simulink subsystem "PID"  (R2024b)
settings: Solver=VariableStepAuto  StartTime=0.0  StopTime=10.0  RelTol=1e-3
values from neighbouring files (symbols this model uses):
  Kd = 1.84    [Controller_PIDTuning.m]
  Ki = 98    [Controller_PIDTuning.m]
  Kp = 32.3    [Controller_PIDTuning.m]
  Kw = 1/Tw    (= 5.88235294118)    [Controller_PIDTuning.m]
  TL = b / wc    [Controller_PIDTuning.m]
settings Model: Creator=Utente  LastModifiedBy=Buton

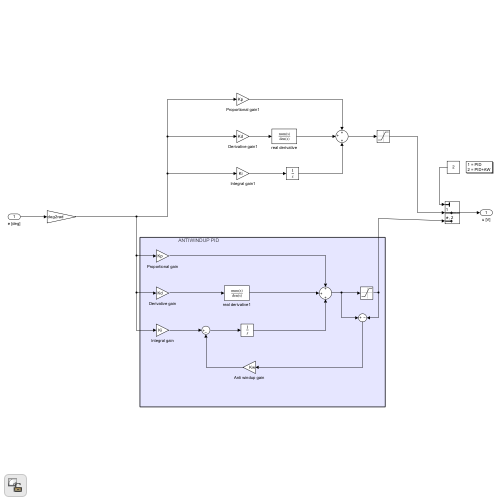
[thumbnail: Simulink's stored preview of the top-level diagram]
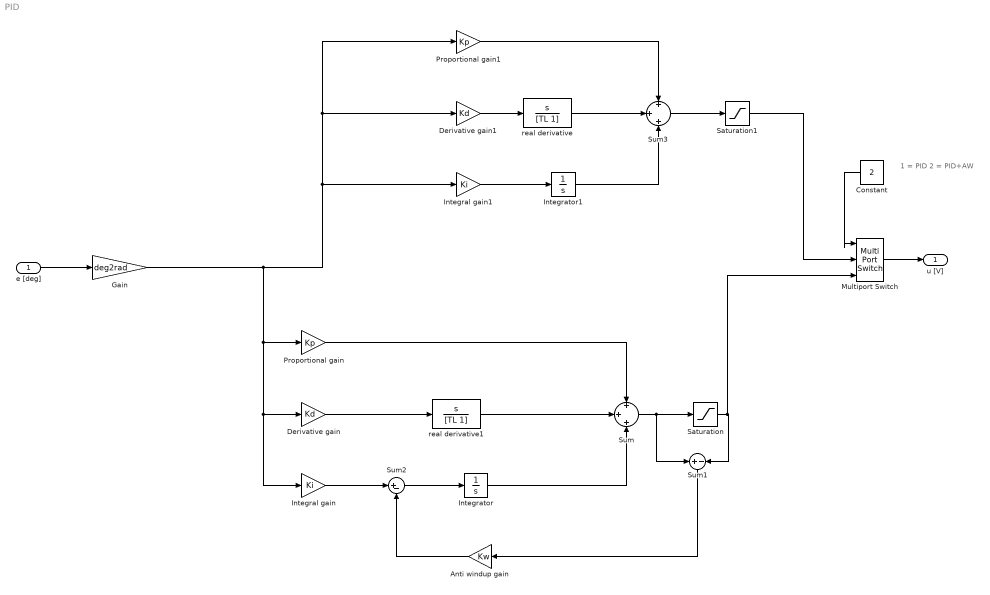
== system PID ==
  note: 1 = PID
      | 2 = PID+AW
  e [deg] : Inport
  Anti windup gain : Gain  Gain=Kw
  Constant : Constant  Value=2
  Derivative gain : Gain  Gain=Kd
  Derivative gain1 : Gain  Gain=Kd
  Gain : Gain  Gain=deg2rad
  Integral gain : Gain  Gain=Ki
  Integral gain1 : Gain  Gain=Ki
  Integrator : Integrator  ZeroCross=off
  Integrator1 : Integrator  ZeroCross=off
  Multiport Switch : MultiPortSwitch  Inputs=2  SaturateOnIntegerOverflow=off  InputSameDT=off
  Proportional gain : Gain  Gain=Kp
  Proportional gain1 : Gain  Gain=Kp
  Saturation : Saturate  UpperLimit=12  LowerLimit=-12
  Saturation1 : Saturate  UpperLimit=10  LowerLimit=-10
  Sum : Sum  Inputs=+|+|+
  Sum1 : Sum  Inputs=+|-
  Sum2 : Sum  Inputs=|+-
  Sum3 : Sum  Inputs=+|+|+
  real derivative : TransferFcn  Numerator=[1 0]  Denominator=[TL 1]
  real derivative1 : TransferFcn  Numerator=[1 0]  Denominator=[TL 1]
  u [V] : Outport
  wires:
  Proportional gain/1 -> Sum/1
  Integrator/1 -> Sum/3
  Derivative gain/1 -> real derivative1/1
  real derivative1/1 -> Sum/2
  Sum/1 -> Sum1/1, Saturation/1
  Saturation/1 -> Sum1/2, Multiport Switch/3
  Sum1/1 -> Anti windup gain/1
  Integral gain/1 -> Sum2/1
  Anti windup gain/1 -> Sum2/2
  Sum2/1 -> Integrator/1
  Sum3/1 -> Saturation1/1
  Proportional gain1/1 -> Sum3/1
  Integrator1/1 -> Sum3/3
  real derivative/1 -> Sum3/2
  Integral gain1/1 -> Integrator1/1
  e [deg]/1 -> Gain/1
  Derivative gain1/1 -> real derivative/1
  Saturation1/1 -> Multiport Switch/2
  Gain/1 -> Proportional gain1/1, Derivative gain1/1, Integral gain1/1, Proportional gain/1, Derivative gain/1, Integral gain/1
  Constant/1 -> Multiport Switch/1
  Multiport Switch/1 -> u [V]/1
